simulink model "decentralized"  (R2023a)
settings: Solver=ode4  StartTime=0.0  StopTime=15  FixedStep=0.001  RelTol=1e-3
values from neighbouring files (symbols this model uses):
  am = [0 inf*9*ones(1,n0) + 0*3.6*(rand(1,n0)-0.5) 0]    [init.m]    (also in init1.m)
  breaktime = 5    [init.m]    (also in init1.m)
  D_ = distance*W(1:n-1,1:n-1)    [init.m]    (also in init1.m)
  g = patch(pp(2,:),pp(1,:),-pp(3,:), v_norm_,'EdgeColor','interp','LineWidth',2)    [demonstration.m]    (also in init.m = 9.8; init1.m = 9.81)
  K = K0    [init.m]    (also in init1.m)
  L0 = ones(n,n)    [init.m]    (also in init1.m)
  M = diag(m)    [init.m]    (also in init1.m)
  M_b = M    [init.m]    (also in init1.m)
  n = n0 + 2    (= 7)    [init.m]    (also in init1.m)
  pp_ = position(:,i)    [demonstration.m]    (also in init.m = [pp_; h0; mass(3)]; init1.m = [pp_; h0; mass(3)])
  v0 = [zeros(1,2+2*(n0+2))]'    [init.m]    (also in init1.m)
  W = ones(n,n)    [init.m]    (also in init1.m)
  W_b = W    [init.m]    (also in init1.m)

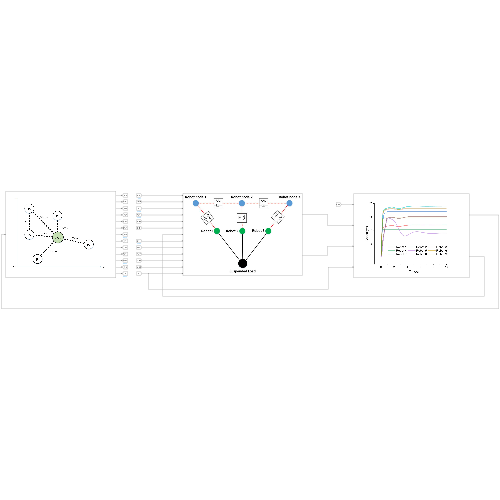
[thumbnail: Simulink's stored preview of the top-level diagram]
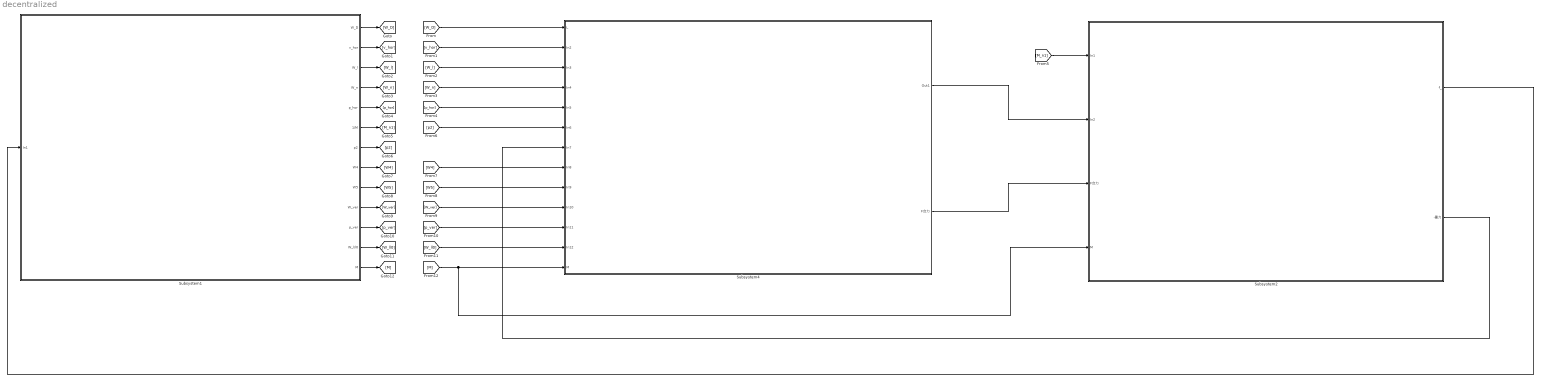
== system decentralized ==
  Subsystem1 : Subsystem
  Subsystem2 : Subsystem
  Subsystem4 : Subsystem
  wires:
  [M_n1] -> Subsystem2/1(In1)
  Subsystem2/1(f_) -> Subsystem1/1(In1)
  [M] -> Subsystem2/4(M), Subsystem4/13(M)
  Subsystem1/1(W_D) -> [W_D]
  Subsystem1/2(v_hor) -> [v_hor]
  Subsystem1/3(W_l) -> [W_l]
  Subsystem1/4(W_n) -> [W_n]
  Subsystem1/5(p_hor) -> [p_hor]
  Subsystem1/6(1/M) -> [M_n1]
  Subsystem1/7(p2) -> [p2]
  Subsystem1/8(W4) -> [W4]
  Subsystem1/9(W5) -> [W5]
  Subsystem1/10(W_ver) -> [W_ver]
  Subsystem1/11(p_ver) -> [p_ver]
  Subsystem1/12(W_l/l0) -> [W_ll0]
  Subsystem1/13(M) -> [M]
  [W_D] -> Subsystem4/1(L)
  [v_hor] -> Subsystem4/2(In2)
  [W_l] -> Subsystem4/3(In3)
  [W_n] -> Subsystem4/4(In4)
  [p_hor] -> Subsystem4/5(In5)
  [p2] -> Subsystem4/6(In6)
  Subsystem2/2(-重力) -> Subsystem4/7(In7)
  [W4] -> Subsystem4/8(In8)
  [W5] -> Subsystem4/9(In9)
  [W_ver] -> Subsystem4/10(In10)
  [p_ver] -> Subsystem4/11(In11)
  [W_ll0] -> Subsystem4/12(In12)
  Subsystem4/1(Out1) -> Subsystem2/2(In2)
  Subsystem4/2(F合力) -> Subsystem2/3(F合力)

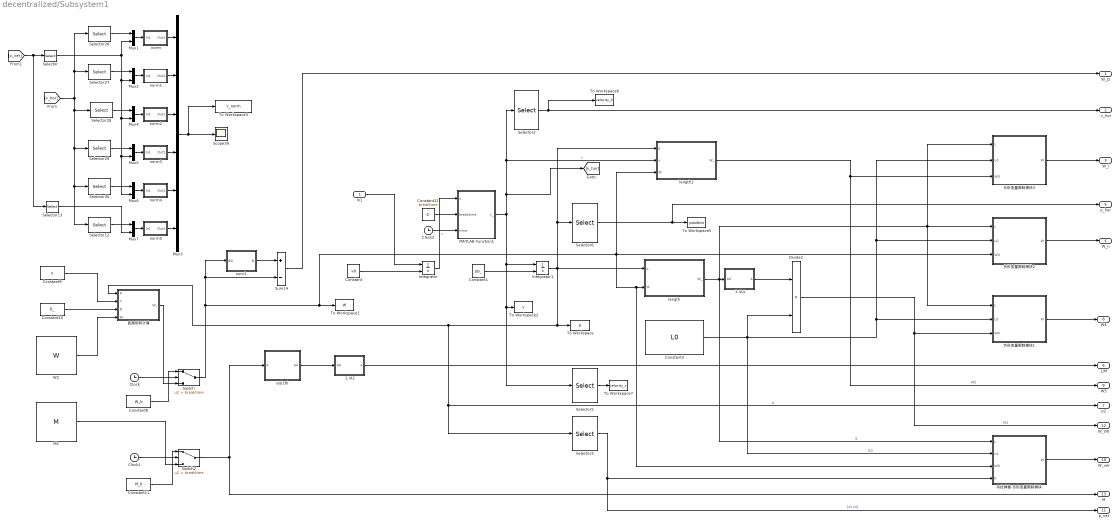
== system decentralized/Subsystem1 ==
  In1 : Inport
  1./A1 : MATLAB Function  TreatAsAtomicUnit=on
  1./A4 : MATLAB Function  TreatAsAtomicUnit=on
  Clock : Clock
  Clock1 : Clock
  Clock2 : Clock
  Constant : Constant  Value=v0
  Constant1 : Constant  Value=pp_
  Constant10 : Constant  Value=D_
  Constant11 : Constant  Value=M_b
  Constant12 : Constant  Value=breaktime
  Constant3 : Constant  Value=L0
  Constant8 : Constant  Value=W_b
  Constant9 : Constant  Value=n
  Divide2 : Product  Inputs=**
  Integrator : Integrator  InitialConditionSource=external
  Integrator1 : Integrator  InitialConditionSource=external
  M3 : Constant  Value=M
  MATLAB Function1 : MATLAB Function  TreatAsAtomicUnit=on
  Mux{1..2,4..7} (6 alike) : Mux  Inputs=2
  Mux3 : Mux  Inputs=6
  Scope39 : Scope
  Selector : Selector  InputPortWidth=2  IndexOptions=Index vector (dialog)  Indices=1  OutputSizes=1
  Selector12 : Selector  InputPortWidth=2*n+2  IndexOptions=Index vector (dialog)  Indices=[13,14]  OutputSizes=1
  Selector13 : Selector  InputPortWidth=2  IndexOptions=Index vector (dialog)  Indices=2  OutputSizes=1
  Selector2 : Selector  InputPortWidth=2*n+2  IndexOptions=Index vector (dialog)  Indices=[1:2*n]  OutputSizes=1
  Selector26 : Selector  InputPortWidth=2*n+2  IndexOptions=Index vector (dialog)  Indices=[3,4]  OutputSizes=1
  Selector27 : Selector  InputPortWidth=2*n+2  IndexOptions=Index vector (dialog)  Indices=[5,6]  OutputSizes=1
  Selector28 : Selector  InputPortWidth=2*n+2  IndexOptions=Index vector (dialog)  Indices=[7,8]  OutputSizes=1
  Selector29 : Selector  InputPortWidth=2*n+2  IndexOptions=Index vector (dialog)  Indices=[9,10]  OutputSizes=1
  Selector3 : Selector  InputPortWidth=2*n+2  IndexOptions=Index vector (dialog)  Indices=[2*n+1 2*n+2]  OutputSizes=1
  Selector30 : Selector  InputPortWidth=2*n+2  IndexOptions=Index vector (dialog)  Indices=[11,12]  OutputSizes=1
  Selector5 : Selector  InputPortWidth=2*n+2  IndexOptions=Index vector (dialog)  Indices=[2*n+1 2*n+2]  OutputSizes=1
  Selector6 : Selector  InputPortWidth=2*n+2  IndexOptions=Index vector (dialog)  Indices=[1:2*n]  OutputSizes=1
  Sum14 : Sum  Inputs=+-
  Switch : Switch  Criteria=u2 > Threshold  Threshold=breaktime  SaturateOnIntegerOverflow=off  InputSameDT=off
  Switch2 : Switch  Criteria=u2 > Threshold  Threshold=breaktime  SaturateOnIntegerOverflow=off  InputSameDT=off
  To Workspace : ToWorkspace  VariableName=p  SaveFormat=Timeseries  SampleTime=-1
  To Workspace1 : ToWorkspace  VariableName=W  SaveFormat=Timeseries  SampleTime=-1
  To Workspace2 : ToWorkspace  VariableName=v  SaveFormat=Timeseries  SampleTime=-1
  To Workspace3 : ToWorkspace  VariableName=v_norm  SaveFormat=Timeseries  SampleTime=-1
  To Workspace5 : ToWorkspace  VariableName=position  SaveFormat=Timeseries  SampleTime=-1
  To Workspace6 : ToWorkspace  VariableName=velocity_h  SaveFormat=Timeseries  SampleTime=-1
  To Workspace7 : ToWorkspace  VariableName=velocity_v  SaveFormat=Timeseries  SampleTime=-1
  W2 : Constant  Value=W
  eq(18) : MATLAB Function  TreatAsAtomicUnit=on
  length : MATLAB Function  TreatAsAtomicUnit=on
  length1 : MATLAB Function  TreatAsAtomicUnit=on
  norm : Subsystem
  norm1 : Subsystem
  norm2 : Subsystem
  norm3 : Subsystem
  norm4 : Subsystem
  norm5 : Subsystem
  sum1 : MATLAB Function  TreatAsAtomicUnit=on
  吊挂弹簧-负形变量限制模块 : MATLAB Function  TreatAsAtomicUnit=on
  负形变量限制模块1 : MATLAB Function  TreatAsAtomicUnit=on
  负形变量限制模块2 : MATLAB Function  TreatAsAtomicUnit=on
  负形变量限制模块3 : MATLAB Function  TreatAsAtomicUnit=on
  距离矩阵计算 : MATLAB Function  TreatAsAtomicUnit=on
  W_D : Outport
  v_hor : Outport  Port=2
  W_l : Outport  Port=3
  W_n : Outport  Port=4
  p_hor : Outport  Port=5
  1/M : Outport  Port=6
  p2 : Outport  Port=7
  W4 : Outport  Port=8
  W5 : Outport  Port=9
  W_ver : Outport  Port=10
  p_ver : Outport  Port=11
  W_l/l0 : Outport  Port=12
  M : Outport  Port=13
  wires:
  Selector/1 -> Mux1/2, Mux6/2, Mux5/2, Mux4/2, Mux2/2
  负形变量限制模块2/1(W) -> W_n/1
  Constant9/1 -> 距离矩阵计算/2(n)
  W2/1 -> 距离矩阵计算/4(W)
  Mux3/1 -> To Workspace3/1, Scope39/1
  1./A4/1(A) -> Divide2/1
  MATLAB Function1/1(v_) -> length1/2(v), Selector2/1, [v_hor], To Workspace2/1, Selector5/1, Integrator1/1  "v"
  Mux6/1 -> norm4/1(In1)
  norm3/1(Out1) -> Mux3/4
  length/1(W_) -> 负形变量限制模块3/1(L), 负形变量限制模块1/1(L), 负形变量限制模块2/1(L), 吊挂弹簧-负形变量限制模块/1(L), 1./A4/1(A0)  "l1"
  Integrator/1 -> MATLAB Function1/1(v)  "v"
  Divide2/1 -> W_l/l0/1, 负形变量限制模块1/3(W0)  "W1"
  Mux7/1 -> norm5/1(In1)
  norm1/1(Out1) -> Mux3/2
  Clock2/1 -> MATLAB Function1/3(time)
  Constant/1 -> Integrator/2
  [v_ver] -> Selector13/1, Selector/1
  Constant10/1 -> 距离矩阵计算/3(D)
  Mux1/1 -> norm/1(In1)
  Selector2/1 -> v_hor/1, To Workspace6/1
  Selector6/1 -> To Workspace5/1, p_hor/1
  Constant3/1 -> 负形变量限制模块1/2(L0), 负形变量限制模块3/2(L0), 负形变量限制模块2/2(L0), 吊挂弹簧-负形变量限制模块/2(L0), Divide2/2  "l10"
  length1/1(W_) -> W5/1, 负形变量限制模块3/3(W0)  "W2"
  In1/1 -> Integrator/1
  M3/1 -> Switch2/3
  Constant1/1 -> Integrator1/2
  norm2/1(Out1) -> Mux3/3
  Integrator1/1 -> p2/1, Selector3/1, 距离矩阵计算/1(p), To Workspace/1, length/1(p), length1/1(p), Selector6/1  "p"
  Selector13/1 -> Mux7/2
  Switch/1 -> sum1/1(B0), Sum14/2, 吊挂弹簧-负形变量限制模块/3(W0), length/2(W), 负形变量限制模块2/3(W0), length1/3(W), To Workspace1/1
  Selector3/1 -> p_ver/1, 吊挂弹簧-负形变量限制模块/4(p)  "[z1 z4]"
  Clock1/1 -> Switch2/2
  负形变量限制模块3/1(W) -> W_l/1
  norm4/1(Out1) -> Mux3/5
  eq(18)/1(AA) -> 1./A1/1(A0)
  Selector5/1 -> To Workspace7/1
  Selector26/1 -> Mux1/1
  Constant11/1 -> Switch2/1
  Clock/1 -> Switch/2
  Constant8/1 -> Switch/1
  距离矩阵计算/1(W_) -> Switch/3
  norm/1(Out1) -> Mux3/1
  sum1/1(B) -> Sum14/1
  Selector28/1 -> Mux4/1
  Constant12/1 -> MATLAB Function1/2(breaktime)
  norm5/1(Out1) -> Mux3/6
  Switch2/1 -> M/1, eq(18)/1(A)
  Selector29/1 -> Mux5/1
  负形变量限制模块1/1(W) -> W4/1
  Mux4/1 -> norm2/1(In1)
  [v_hor] -> Selector12/1, Selector30/1, Selector29/1, Selector28/1, Selector26/1, Selector27/1
  Selector30/1 -> Mux6/1
  Mux2/1 -> norm1/1(In1)
  Selector27/1 -> Mux2/1
  Mux5/1 -> norm3/1(In1)
  Selector12/1 -> Mux7/1
  1./A1/1(A) -> 1/M/1
  Sum14/1 -> W_D/1
  吊挂弹簧-负形变量限制模块/1(W) -> W_ver/1

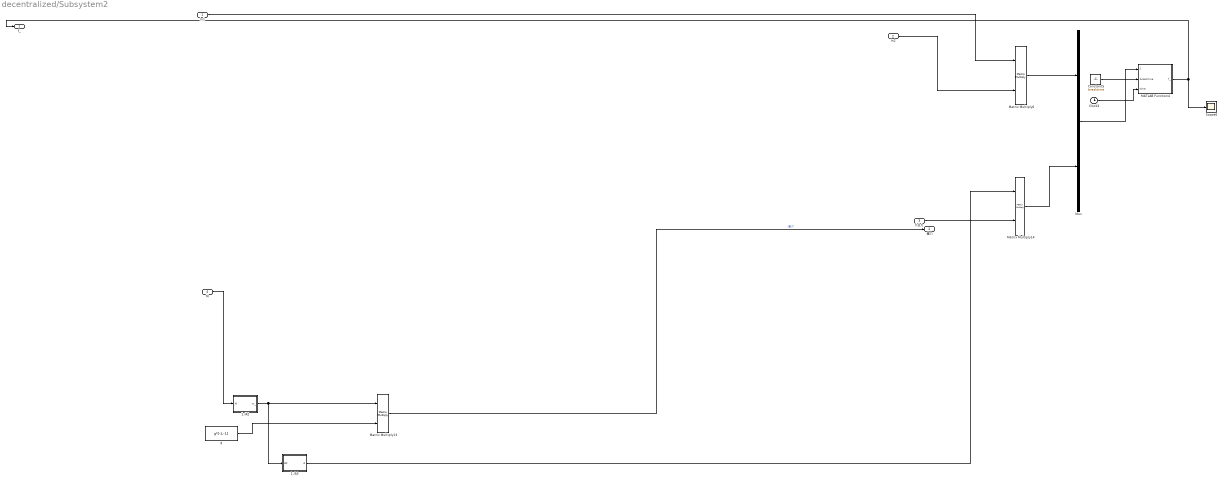
== system decentralized/Subsystem2 ==
  In1 : Inport
  In2 : Inport  Port=2
  F合力 : Inport  Port=3
  M : Inport  Port=4
  1./A2 : MATLAB Function  TreatAsAtomicUnit=on
  1./A3 : MATLAB Function  TreatAsAtomicUnit=on
  Clock3 : Clock
  Constant5 : Constant  Value=breaktime
  MATLAB Function4 : MATLAB Function  TreatAsAtomicUnit=on
  Matrix Multiply13 : Product  Multiplication=Matrix(*)
  Matrix Multiply14 : Product  Multiplication=Matrix(*)
  Matrix Multiply6 : Product  Multiplication=Matrix(*)
  Mux : Mux  Inputs=2
  Scope6 : Scope
  g : Constant  Value=g*[-1;-1]
  f_ : Outport
  -重力 : Outport  Port=2
  wires:
  1./A2/1(m_) -> 1./A3/1(A0), Matrix Multiply13/1
  g/1 -> Matrix Multiply13/2
  M/1 -> 1./A2/1(M)
  1./A3/1(A) -> Matrix Multiply14/1
  MATLAB Function4/1(f_) -> f_/1, Scope6/1
  Clock3/1 -> MATLAB Function4/3(time)
  Matrix Multiply6/1 -> Mux/1
  Constant5/1 -> MATLAB Function4/2(breaktime)
  Matrix Multiply14/1 -> Mux/2
  Mux/1 -> MATLAB Function4/1(f)
  F合力/1 -> Matrix Multiply14/2
  In1/1 -> Matrix Multiply6/1
  In2/1 -> Matrix Multiply6/2
  Matrix Multiply13/1 -> -重力/1  "-重力"

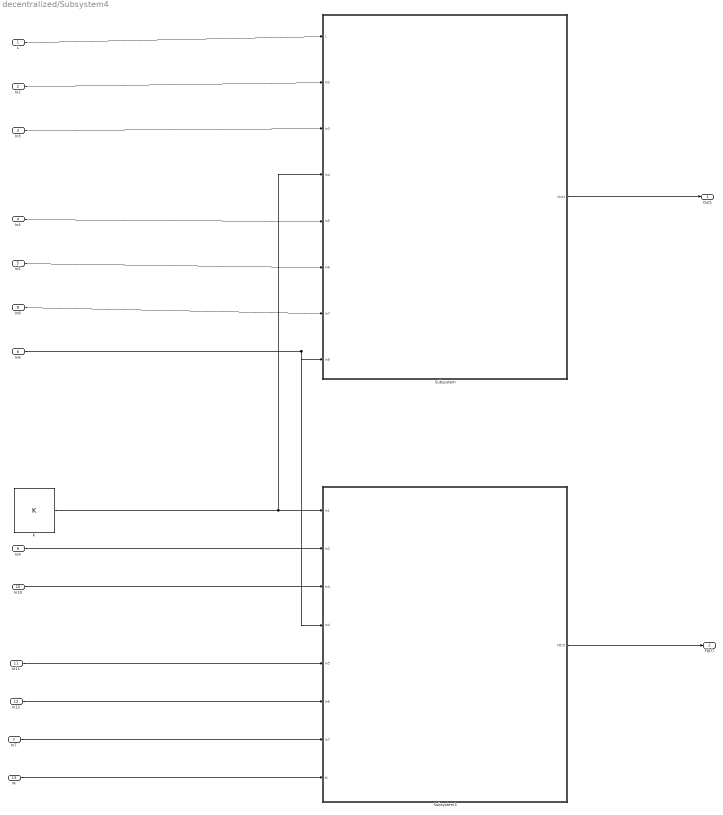
== system decentralized/Subsystem4 ==
  L : Inport
  In2 : Inport  Port=2
  In3 : Inport  Port=3
  In4 : Inport  Port=4
  In5 : Inport  Port=5
  In6 : Inport  Port=6
  In7 : Inport  Port=7
  In8 : Inport  Port=8
  In9 : Inport  Port=9
  In10 : Inport  Port=10
  In11 : Inport  Port=11
  In12 : Inport  Port=12
  M : Inport  Port=13
  K : Constant  Value=K
  Subsystem : Subsystem
  Subsystem3 : Subsystem
  Out1 : Outport
  F合力 : Outport  Port=2
  wires:
  In2/1 -> Subsystem/2(In2)
  K/1 -> Subsystem/4(In4), Subsystem3/1(In1)
  In10/1 -> Subsystem3/3(In3)
  In5/1 -> Subsystem/6(In6)
  M/1 -> Subsystem3/8(M)
  In6/1 -> Subsystem/8(In8), Subsystem3/4(In4)
  In9/1 -> Subsystem3/2(In2)
  In4/1 -> Subsystem/5(In5)
  L/1 -> Subsystem/1(L)
  In11/1 -> Subsystem3/5(In5)
  Subsystem3/1(F合力) -> F合力/1
  Subsystem/1(Out1) -> Out1/1
  In7/1 -> Subsystem3/7(In7)
  In8/1 -> Subsystem/7(In7)
  In12/1 -> Subsystem3/6(In6)
  In3/1 -> Subsystem/3(In3)

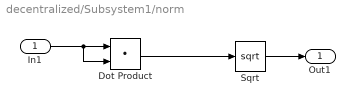
== system decentralized/Subsystem1/norm ==
  In1 : Inport
  Dot Product : DotProduct  OutDataTypeStr=Inherit: Inherit via internal rule
  Sqrt : Sqrt
  Out1 : Outport
  wires:
  In1/1 -> Dot Product/2, Dot Product/1
  Dot Product/1 -> Sqrt/1
  Sqrt/1 -> Out1/1

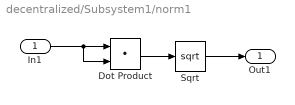
== system decentralized/Subsystem1/norm1 ==
  In1 : Inport
  Dot Product : DotProduct  OutDataTypeStr=Inherit: Inherit via internal rule
  Sqrt : Sqrt
  Out1 : Outport
  wires:
  Sqrt/1 -> Out1/1
  Dot Product/1 -> Sqrt/1
  In1/1 -> Dot Product/1, Dot Product/2

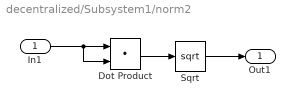
== system decentralized/Subsystem1/norm2 ==
  In1 : Inport
  Dot Product : DotProduct  OutDataTypeStr=Inherit: Inherit via internal rule
  Sqrt : Sqrt
  Out1 : Outport
  wires:
  In1/1 -> Dot Product/2, Dot Product/1
  Dot Product/1 -> Sqrt/1
  Sqrt/1 -> Out1/1

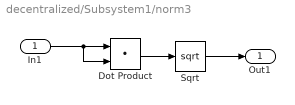
== system decentralized/Subsystem1/norm3 ==
  In1 : Inport
  Dot Product : DotProduct  OutDataTypeStr=Inherit: Inherit via internal rule
  Sqrt : Sqrt
  Out1 : Outport
  wires:
  Sqrt/1 -> Out1/1
  Dot Product/1 -> Sqrt/1
  In1/1 -> Dot Product/1, Dot Product/2

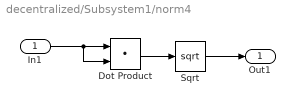
== system decentralized/Subsystem1/norm4 ==
  In1 : Inport
  Dot Product : DotProduct  OutDataTypeStr=Inherit: Inherit via internal rule
  Sqrt : Sqrt
  Out1 : Outport
  wires:
  In1/1 -> Dot Product/2, Dot Product/1
  Dot Product/1 -> Sqrt/1
  Sqrt/1 -> Out1/1

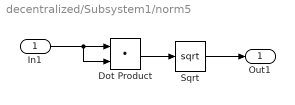
== system decentralized/Subsystem1/norm5 ==
  In1 : Inport
  Dot Product : DotProduct  OutDataTypeStr=Inherit: Inherit via internal rule
  Sqrt : Sqrt
  Out1 : Outport
  wires:
  Sqrt/1 -> Out1/1
  Dot Product/1 -> Sqrt/1
  In1/1 -> Dot Product/1, Dot Product/2

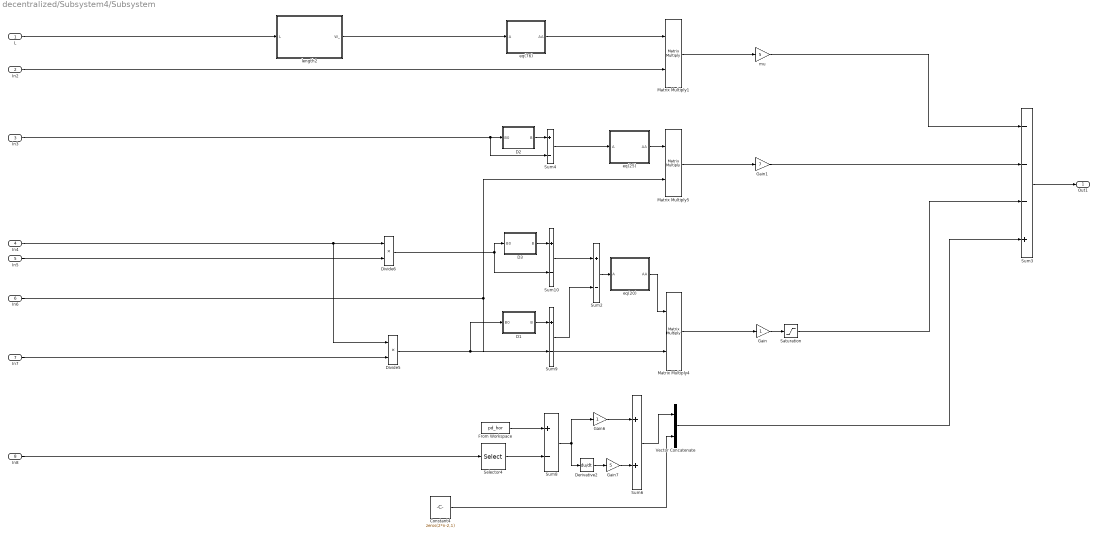
== system decentralized/Subsystem4/Subsystem ==
  L : Inport
  In2 : Inport  Port=2
  In3 : Inport  Port=3
  In4 : Inport  Port=4
  In5 : Inport  Port=5
  In6 : Inport  Port=6
  In7 : Inport  Port=7
  In8 : Inport  Port=8
  Constant4 : Constant  Value=zeros(2*n-2,1)
  D1 : MATLAB Function  TreatAsAtomicUnit=on
  D2 : MATLAB Function  TreatAsAtomicUnit=on
  D3 : MATLAB Function  TreatAsAtomicUnit=on
  Derivative2 : Derivative
  Divide5 : Product  Inputs=**
  Divide6 : Product  Inputs=**
  From Workspace : FromWorkspace  VariableName=pd_hor
  Gain : Gain
  Gain1 : Gain  Gain=7
  Gain6 : Gain
  Gain7 : Gain  Gain=5
  Matrix Multiply1 : Product  Multiplication=Matrix(*)
  Matrix Multiply4 : Product  Multiplication=Matrix(*)
  Matrix Multiply5 : Product  Multiplication=Matrix(*)
  Saturation : Saturate  UpperLimit=100  LowerLimit=-100
  Selector4 : Selector  InputPortWidth=2*n+2  IndexOptions=Index vector (dialog)  Indices=[1 2]  OutputSizes=1
  Sum{2,4,8..10} (5 alike) : Sum  Inputs=+-
  Sum3 : Sum  Inputs=---+
  Sum6 : Sum
  Vector Concatenate : Concatenate
  eq(20) : MATLAB Function  TreatAsAtomicUnit=on
  eq(25) : MATLAB Function  TreatAsAtomicUnit=on
  eq(76) : MATLAB Function  TreatAsAtomicUnit=on
  length2 : MATLAB Function  TreatAsAtomicUnit=on
  mu : Gain  Gain=5
  Out1 : Outport
  wires:
  Derivative2/1 -> Gain7/1
  In3/1 -> Sum4/2, D2/1(B0)
  Sum4/1 -> eq(25)/1(A)
  L/1 -> length2/1(L)
  In6/1 -> Matrix Multiply5/2, Matrix Multiply4/2
  Gain6/1 -> Sum6/1
  Sum9/1 -> Sum2/2
  D2/1(B) -> Sum4/1
  Saturation/1 -> Sum3/3
  Gain1/1 -> Sum3/2
  Selector4/1 -> Sum8/2
  D3/1(B) -> Sum10/1
  Sum8/1 -> Gain6/1, Derivative2/1
  Divide5/1 -> Sum9/2, D1/1(B0)
  eq(76)/1(AA) -> Matrix Multiply1/1
  Sum2/1 -> eq(20)/1(A)
  Gain7/1 -> Sum6/2
  Sum3/1 -> Out1/1
  Vector Concatenate/1 -> Sum3/4
  eq(25)/1(AA) -> Matrix Multiply5/1
  Divide6/1 -> Sum10/2, D3/1(B0)
  Matrix Multiply1/1 -> mu/1
  In8/1 -> Selector4/1
  In2/1 -> Matrix Multiply1/2
  mu/1 -> Sum3/1
  Constant4/1 -> Vector Concatenate/2
  D1/1(B) -> Sum9/1
  Matrix Multiply5/1 -> Gain1/1
  Matrix Multiply4/1 -> Gain/1
  From Workspace/1 -> Sum8/1
  length2/1(W_) -> eq(76)/1(A)
  Sum10/1 -> Sum2/1
  In4/1 -> Divide5/1, Divide6/1
  In7/1 -> Divide5/2
  eq(20)/1(AA) -> Matrix Multiply4/1
  Sum6/1 -> Vector Concatenate/1
  Gain/1 -> Saturation/1
  In5/1 -> Divide6/2

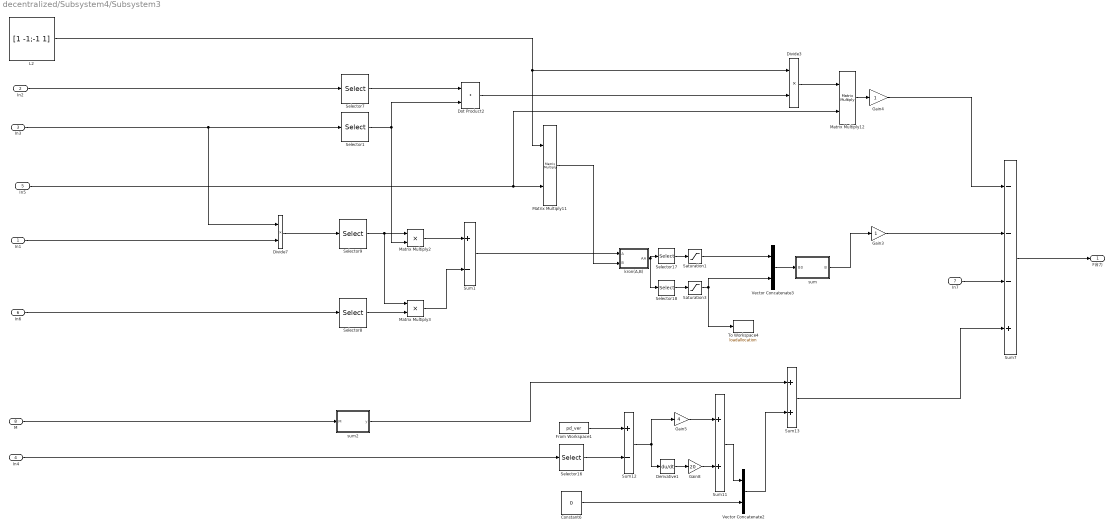
== system decentralized/Subsystem4/Subsystem3 ==
  In1 : Inport
  In2 : Inport  Port=2
  In3 : Inport  Port=3
  In4 : Inport  Port=4
  In5 : Inport  Port=5
  In6 : Inport  Port=6
  In7 : Inport  Port=7
  M : Inport  Port=8
  Constant6 : Constant  Value=0
  Derivative1 : Derivative
  Divide3 : Product  Inputs=**
  Divide7 : Product  Inputs=**
  Dot Product2 : DotProduct  OutDataTypeStr=Inherit: Inherit via internal rule
  From Workspace1 : FromWorkspace  VariableName=pd_ver
  Gain3 : Gain
  Gain4 : Gain
  Gain5 : Gain  Gain=4
  Gain8 : Gain  Gain=20
  L2 : Constant  Value=[1 -1;-1 1]
  Matrix Multiply11 : Product  Multiplication=Matrix(*)
  Matrix Multiply12 : Product  Multiplication=Matrix(*)
  Matrix Multiply2 : Product
  Matrix Multiply3 : Product
  Saturation1 : Saturate  UpperLimit=am  LowerLimit=-am
  Saturation3 : Saturate  UpperLimit=am  LowerLimit=-am
  Selector{1,7..9} (4 alike) : Selector  NumberOfDimensions=2  InputPortWidth=6  IndexOptions=Index vector (dialog),Index vector (dialog)  Indices=n,[1:n]  OutputSizes=1,1
  Selector16 : Selector  InputPortWidth=2*n+2  IndexOptions=Index vector (dialog)  Indices=2*n+1  OutputSizes=1
  Selector17 : Selector  NumberOfDimensions=2  InputPortWidth=6  IndexOptions=Index vector (dialog),Index vector (dialog)  Indices=1,[1:n]  OutputSizes=1,1
  Selector18 : Selector  NumberOfDimensions=2  InputPortWidth=6  IndexOptions=Index vector (dialog),Index vector (dialog)  Indices=2,[1:n]  OutputSizes=1,1
  Sum1 : Sum  Inputs=+-
  Sum11 : Sum
  Sum12 : Sum  Inputs=+-
  Sum13 : Sum
  Sum7 : Sum  Inputs=---+
  To Workspace4 : ToWorkspace  VariableName=loadallocation  SaveFormat=Timeseries  SampleTime=-1
  Vector Concatenate2 : Concatenate
  Vector Concatenate3 : Concatenate  Mode=Multidimensional array
  kron(A,B) : MATLAB Function  TreatAsAtomicUnit=on
  sum : MATLAB Function  TreatAsAtomicUnit=on
  sum2 : MATLAB Function  TreatAsAtomicUnit=on
  F合力 : Outport
  wires:
  Divide7/1 -> Selector9/1
  Selector8/1 -> Matrix Multiply3/2
  In1/1 -> Divide7/2
  Selector7/1 -> Dot Product2/1
  Gain8/1 -> Sum11/2
  In2/1 -> Selector7/1
  Sum12/1 -> Gain5/1, Derivative1/1
  Sum11/1 -> Vector Concatenate2/1
  In3/1 -> Divide7/1, Selector1/1
  L2/1 -> Matrix Multiply11/1, Divide3/1
  Matrix Multiply11/1 -> kron(A,B)/2(B)
  In5/1 -> Matrix Multiply12/2, Matrix Multiply11/2
  Gain4/1 -> Sum7/1
  Saturation3/1 -> To Workspace4/1, Vector Concatenate3/2
  From Workspace1/1 -> Sum12/1
  Derivative1/1 -> Gain8/1
  Dot Product2/1 -> Divide3/2
  Selector9/1 -> Matrix Multiply2/1, Matrix Multiply3/1
  Selector18/1 -> Saturation3/1
  Selector1/1 -> Dot Product2/2, Matrix Multiply2/2
  Sum1/1 -> kron(A,B)/1(A)
  sum2/1(y) -> Sum13/1
  kron(A,B)/1(AA) -> Selector17/1, Selector18/1
  Gain3/1 -> Sum7/2
  Matrix Multiply2/1 -> Sum1/1
  Selector16/1 -> Sum12/2
  Constant6/1 -> Vector Concatenate2/2
  Saturation1/1 -> Vector Concatenate3/1
  Vector Concatenate3/1 -> sum/1(B0)
  In7/1 -> Sum7/3
  sum/1(B) -> Gain3/1
  Matrix Multiply12/1 -> Gain4/1
  Matrix Multiply3/1 -> Sum1/2
  Gain5/1 -> Sum11/1
  In6/1 -> Selector8/1
  Selector17/1 -> Saturation1/1
  Sum7/1 -> F合力/1
  In4/1 -> Selector16/1
  Divide3/1 -> Matrix Multiply12/1
  Vector Concatenate2/1 -> Sum13/2
  Sum13/1 -> Sum7/4
  M/1 -> sum2/1(M)

== matlab function decentralized/Subsystem4/Subsystem/eq(76) ==
function AA = fcn(A)
I = eye(2);
AA = kron(A,I);

== matlab function decentralized/Subsystem1/吊挂弹簧-负形变量限制模块 ==
function W = fcn(L,L0,W0,p)
    [m,n] = size(L);
    W = zeros(m,n);
    for i = 1:m
        for j = 1:n
            if i==m || j==n
                if L(i,j)<L0(i,j) || p(1)>p(2) %现长<原长 重物高度比托盘高度高
                    W(i,j) = 0;
                    %W(i,j) = W0(i,j);
                else
                    %W(i,j) = 0;
                    W(i,j) = W0(i,j);
                end
            else 
                    W(i,j) = W0(i,j);
            end
        end
    end
end

== matlab function decentralized/Subsystem1/负形变量限制模块1 ==
function W = fcn(L,L0,W0)
    [m,n] = size(L);
    W = zeros(m,n);
    for i = 1:m
        for j = 1:n
            if i==m || j==n
                if L(i,j)<L0(i,j)
                    W(i,j) = 0;
                else
                    W(i,j) = W0(i,j);
                end
            else 
                    W(i,j) = W0(i,j);
            end
        end
    end
end

== matlab function decentralized/Subsystem4/Subsystem/D3 ==
function B = fcn(B0)
[m,n] = size(B0);
B = zeros(m,m);
for i = 1:m
    B(i,i) = sum(B0(i,:)); 
end

== matlab function decentralized/Subsystem1/负形变量限制模块2 ==
function W = fcn(L,L0,W0)
    [m,n] = size(L);
    W = zeros(m,n);
    for i = 1:m
        for j = 1:n
            if i==m || j==n
                if L(i,j)<L0(i,j)
                    W(i,j) = 0;
                else
                    W(i,j) = W0(i,j);
                end
            else 
                    W(i,j) = W0(i,j);
            end
        end
    end
end

== matlab function decentralized/Subsystem1/负形变量限制模块3 ==
function W = fcn(L,L0,W0)
    [m,n] = size(L);
    W = zeros(m,n);
    for i = 1:m
        for j = 1:n
            if i==m || j==n
                if L(i,j)<L0(i,j)
                    W(i,j) = 0;
                else
                    W(i,j) = W0(i,j);
                end
            else 
                    W(i,j) = W0(i,j);
            end
        end
    end
end

== matlab function decentralized/Subsystem2/MATLAB Function4 ==
function f_ = fcn(f, breaktime,time)
%     [m,n] = size(f);% 10行1列
    f_ = f;
    if time > breaktime
            f_([9:12]) = zeros(4,1);
    end
end

== matlab function decentralized/Subsystem4/Subsystem3/kron(A,B) ==
function AA = fcn(A,B)
% I = ones(2,1);
AA = kron(A,B);
end

== matlab function decentralized/Subsystem4/Subsystem3/sum ==
function B = fcn(B0)
B = sum(B0,2); 
end

== matlab function decentralized/Subsystem1/距离矩阵计算 ==
function W_ = fcn(p,n,D,W)
%     D = L0(1:n-1, 1:n-1); %感知范围矩阵
% 循环计算两个点之间的距离
    W_ = W;
    for i = 1:n-1
        for j = 1:n-1
            d = norm([p(2*i-1);p(2*i);p(end-1)] - [p(2*j-1);p(2*j);p(end-1)],2);
            if d > D(i,j)
                W_(i,j) = 0;
            end
        end
    end
end

== matlab function decentralized/Subsystem1/sum1 ==
function B = fcn(B0)
[m,n] = size(B0);
B = zeros(m,n);
for i = 1:m
    B(i,i) = sum(B0(i,:)); 
end
end

== matlab function decentralized/Subsystem2/1.//A2 ==
function m_ = fcn(M)
    m = diag(M);
    m_ = [sum(m(1:end-1)) 0;0 m(end)];
end

== matlab function decentralized/Subsystem1/MATLAB Function1 ==
function v_ = fcn(v, breaktime, time)
    v_ = v;
    if time >= breaktime
        v_([9,10,11,12]) = zeros(1,4);
    end
end

== matlab function decentralized/Subsystem4/Subsystem3/sum2 ==
function y = fcn(M)
    g = 9.8;
    y = [-trace(M)*g; 0]; 
end

== matlab function decentralized/Subsystem1/length ==
function W_ = fcn(p,W)
l = size(p,1);
[m,n] = size(W);
W_ = zeros(m,n);
p_ = zeros(3,m);
for kk = 1:m
    if kk == m
        p_(:,kk) = [p(2*kk-1);p(2*kk);p(l)];
    else
        p_(:,kk) = [p(2*kk-1);p(2*kk);p(l-1)];
    end
end
for i = 1:m
    for j = 1:n
        if W(i,j) == 0
            W_(i,j) = 0;
        else
            W_(i,j) = norm((p_(:,i) - p_(:,j)),2);
        end
    end
end

== matlab function decentralized/Subsystem4/Subsystem/length2 ==
function W_ = fcn(L)
[m,n] = size(L);
W_ = zeros(m,n);

for i = 1:m
    for j = 1:n
        if i == 1 || j==1
            W_(i,j) = L(i,j);
        else if i==j
            W_(i,j) = 1;
        end
        if i==j & i==m
            W_(i,j) = 0;
        end
        end
    end
end

== matlab function decentralized/Subsystem1/1.//A4 ==
function A = fcn(A0)
[m,n] = size(A0);
A = zeros(m,n);
for i = 1:m
    for j = 1:n
        if A0(i,j) == 0;
            A(i,j) = 0;
        else
            A(i,j) = 1/A0(i,j);
        end
    end
end

== matlab function decentralized/Subsystem1/1.//A1 ==
function A = fcn(A0)
[m,n] = size(A0);
A = zeros(m,n);
for i = 1:m
    for j = i:n
        if A0(i,j) == 0;
            A(i,j) = 0;
        else
            A(i,j) = 1/A0(i,j);
        end
    end
end

== matlab function decentralized/Subsystem1/length1 ==
function W_ = fcn(p,v,W)
l = size(p,1);
[m,n] = size(W);
W_ = zeros(m,n);
p_ = zeros(3,m);
v_ = zeros(3,m);
for kk = 1:m
    if kk == m
        p_(:,kk) = [p(2*kk-1);p(2*kk);p(l)];
        v_(:,kk) = [v(2*kk-1);v(2*kk);v(l)];
    else
        p_(:,kk) = [p(2*kk-1);p(2*kk);p(l-1)];
        v_(:,kk) = [v(2*kk-1);v(2*kk);v(l-1)];
    end
end

for i = 1:m
    for j = 1:n
        if W(i,j) == 0
            W_(i,j) = 0;
        else
            W_(i,j) = dot((p_(:,i) - p_(:,j)),(v_(:,i) - v_(:,j)))/(norm((p_(:,i) - p_(:,j)),2))^2;
        end
    end
end

== matlab function decentralized/Subsystem4/Subsystem/D2 ==
function B = fcn(B0)
[m,n] = size(B0);
B = zeros(m,m);
for i = 1:m
    B(i,i) = sum(B0(i,:)); 
end

== matlab function decentralized/Subsystem1/eq(18) ==
function AA = fcn(A)
I = eye(2);
AA = kron(A,I);

== matlab function decentralized/Subsystem2/1.//A3 ==
function A = fcn(A0)
[m,n] = size(A0);
A = zeros(m,n);
for i = 1:m
    for j = i:n
        if A0(i,j) == 0;
            A(i,j) = 0;
        else
            A(i,j) = 1/A0(i,j);
        end
    end
end

== matlab function decentralized/Subsystem4/Subsystem/eq(20) ==
function AA = fcn(A)
I = eye(2);
AA = kron(A,I);

== matlab function decentralized/Subsystem4/Subsystem/eq(25) ==
function AA = fcn(A)
I = eye(2);
AA = kron(A,I);

== matlab function decentralized/Subsystem4/Subsystem/D1 ==
function B = fcn(B0)
[m,n] = size(B0);
B = zeros(m,m);
for i = 1:m
    B(i,i) = sum(B0(i,:)); 
end
